simulink model "Day1_model3"  (R2022b)
settings: Solver=ode4  StartTime=0.0  StopTime=10.0  FixedStep=0.001  RelTol=1e-3
values from neighbouring files (symbols this model uses):
  D = 3    [Day1.m]    (also in Day1_3.m = 1)
  K = 10    [Day1.m]    (also in Day1_3.m)
  Kd = 500    [Day1_3.m]
  Kp = 10000    [Day1_3.m]
  M = 1    [Day1.m]    (also in Day1_3.m = 10)
settings Model: Creator=user  LastModifiedBy=user

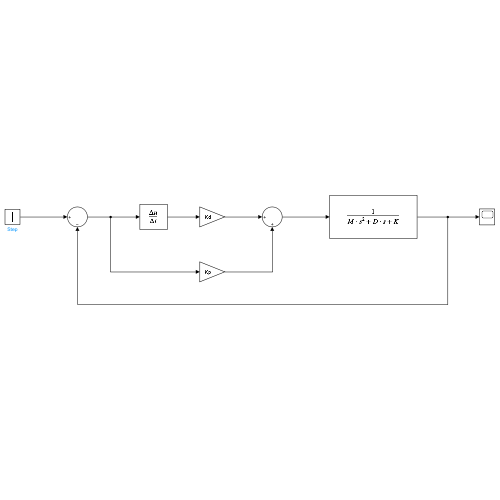
[thumbnail: Simulink's stored preview of the top-level diagram]
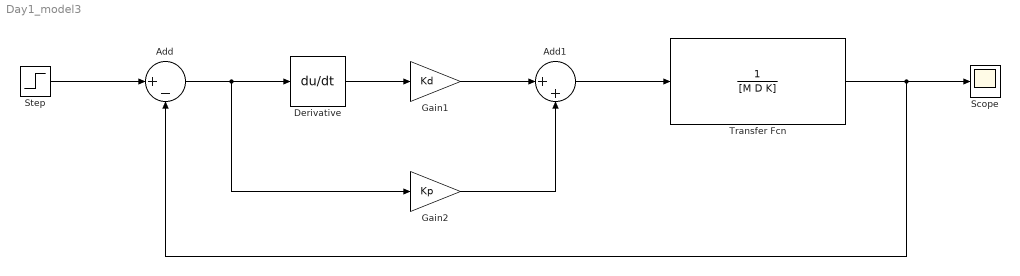
== system Day1_model3 ==
  Add : Sum  Inputs=|+-
  Add1 : Sum  Inputs=|++
  Derivative : Derivative
  Gain1 : Gain  Gain=Kd
  Gain2 : Gain  Gain=Kp
  Scope : Scope
  Step : Step  SampleTime=0
  Transfer Fcn : TransferFcn  Denominator=[M D K]
  wires:
  Transfer Fcn/1 -> Add/2, Scope/1
  Step/1 -> Add/1
  Add/1 -> Gain2/1, Derivative/1
  Derivative/1 -> Gain1/1
  Gain1/1 -> Add1/1
  Add1/1 -> Transfer Fcn/1
  Gain2/1 -> Add1/2
